simulink model "PX4_Run_Mode_R2017b"  (R2017b)
settings: Solver=FixedStepDiscrete  StartTime=0.0  StopTime=10.0  RelTol=1e-3  EnableMultiTasking=on
InitFcn:
  | run('InitFcn_R2017b_no_csc.m');
values from neighbouring files (symbols this model uses):
  A = Pixhawk_CSC.Parameter( {single([diag([1 1 1]) Ts*diag([1 1 1]); diag([0 0 0]) diag([1 1 1])]),'A'} )    [InitFcn.m]    (also in InitFcn_R2016b.m; InitFcn_R2017b_no_csc.m = single([diag([1 1 1]) Ts*diag([1 1 1]); diag([0 0 0]) diag([)
  app = Pixhawk_CSC.Parameter({single( [0.05; 0.05; 0.05]),'app'} )    [InitFcn.m]    (also in InitFcn_R2016b.m; InitFcn_R2017b_no_csc.m = single( [0.05; 0.05; 0.05]))
  B = Pixhawk_CSC.Parameter( {single([Ts^2/2*diag([1 1 1]); Ts*diag([1 1 1])]),'B'} )    [InitFcn.m]    (also in InitFcn_R2016b.m; InitFcn_R2017b_no_csc.m = single([Ts^2/2*diag([1 1 1]); Ts*diag([1 1 1])]))
  Beta = Pixhawk_CSC.Parameter({single( 0.02),'Beta'} )    [InitFcn.m]    (also in InitFcn_R2016b.m; InitFcn_R2017b_no_csc.m = single( 0.02))
  C = Pixhawk_CSC.Parameter( {single([diag([1 1 1]) 0*diag([1 1 1]); zeros(1,2) 1 zeros(1,3)]),'C'} )    [InitFcn.m]    (also in InitFcn_R2016b.m; InitFcn_R2017b_no_csc.m = single([diag([1 1 1]) 0*diag([1 1 1]); zeros(1,2) 1 zeros(1,)
  C1 = Pixhawk_CSC.Parameter({single( 1.08680),'C1'} )    [InitFcn.m]    (also in InitFcn_R2016b.m; InitFcn_R2017b_no_csc.m = single( 1.08680))
  C10 = Pixhawk_CSC.Parameter({single( 0.0000),'C10'} )    [InitFcn.m]    (also in InitFcn_R2016b.m; InitFcn_R2017b_no_csc.m = single( 0.0000))
  C11 = Pixhawk_CSC.Parameter({single(-0.2300),'C11'} )    [InitFcn.m]    (also in InitFcn_R2016b.m; InitFcn_R2017b_no_csc.m = single(-0.2300))
  C12 = Pixhawk_CSC.Parameter({single( 0.0000),'C12'} )    [InitFcn.m]    (also in InitFcn_R2016b.m; InitFcn_R2017b_no_csc.m = single( 0.0000))
  C13 = Pixhawk_CSC.Parameter({single( 0.8000),'C13'} )    [InitFcn.m]    (also in InitFcn_R2016b.m; InitFcn_R2017b_no_csc.m = single( 0.8000))
  C14 = Pixhawk_CSC.Parameter({single( 0.8000),'C14'} )    [InitFcn.m]    (also in InitFcn_R2016b.m; InitFcn_R2017b_no_csc.m = single( 0.8000))
  C15 = Pixhawk_CSC.Parameter({single( 1.73200),'C15'} )    [InitFcn.m]    (also in InitFcn_R2016b.m; InitFcn_R2017b_no_csc.m = single( 1.73200))
  C16 = Pixhawk_CSC.Parameter({single( 0.1000),'C16'} )    [InitFcn.m]    (also in InitFcn_R2016b.m; InitFcn_R2017b_no_csc.m = single( 0.1000))
  C17 = Pixhawk_CSC.Parameter({single( 0.1000),'C17'} )    [InitFcn.m]    (also in InitFcn_R2016b.m; InitFcn_R2017b_no_csc.m = single( 0.1000))
  C18 = Pixhawk_CSC.Parameter({single( 0.0500),'C18'} )    [InitFcn.m]    (also in InitFcn_R2016b.m; InitFcn_R2017b_no_csc.m = single( 0.0500))
  C19 = Pixhawk_CSC.Parameter({single( 0.6000),'C19'} )    [InitFcn.m]    (also in InitFcn_R2016b.m; InitFcn_R2017b_no_csc.m = single( 0.6000))
  C2 = Pixhawk_CSC.Parameter({single( 1.10468),'C2'} )    [InitFcn.m]    (also in InitFcn_R2016b.m; InitFcn_R2017b_no_csc.m = single( 1.10468))
  C20 = Pixhawk_CSC.Parameter({single( 0.6000),'C20'} )    [InitFcn.m]    (also in InitFcn_R2016b.m; InitFcn_R2017b_no_csc.m = single( 0.6000))
  C21 = Pixhawk_CSC.Parameter({single( 1.04558),'C21'} )    [InitFcn.m]    (also in InitFcn_R2016b.m; InitFcn_R2017b_no_csc.m = single( 1.04558))
  C22 = Pixhawk_CSC.Parameter({single( 0.0000),'C22'} )    [InitFcn.m]    (also in InitFcn_R2016b.m; InitFcn_R2017b_no_csc.m = single( 0.0000))
  C23 = Pixhawk_CSC.Parameter({single( 0.0000),'C23'} )    [InitFcn.m]    (also in InitFcn_R2016b.m; InitFcn_R2017b_no_csc.m = single( 0.0000))
  C24 = Pixhawk_CSC.Parameter({single(-11.0000),'C24'} )    [InitFcn.m]    (also in InitFcn_R2016b.m; InitFcn_R2017b_no_csc.m = single(-11.0000))
  C3 = Pixhawk_CSC.Parameter({single( 1.1980),'C3'} )    [InitFcn.m]    (also in InitFcn_R2016b.m; InitFcn_R2017b_no_csc.m = single( 1.1980))
  C4 = Pixhawk_CSC.Parameter({single( 0.0500),'C4'} )    [InitFcn.m]    (also in InitFcn_R2016b.m; InitFcn_R2017b_no_csc.m = single( 0.0500))
  C5 = Pixhawk_CSC.Parameter({single( 0.0500),'C5'} )    [InitFcn.m]    (also in InitFcn_R2016b.m; InitFcn_R2017b_no_csc.m = single( 0.0500))
  C6 = Pixhawk_CSC.Parameter({single( 0.0500),'C6'} )    [InitFcn.m]    (also in InitFcn_R2016b.m; InitFcn_R2017b_no_csc.m = single( 0.0500))
  C7 = Pixhawk_CSC.Parameter({single( 0.35937),'C7'} )    [InitFcn.m]    (also in InitFcn_R2016b.m; InitFcn_R2017b_no_csc.m = single( 0.35937))
  C8 = Pixhawk_CSC.Parameter({single( 0.36528),'C8'} )    [InitFcn.m]    (also in InitFcn_R2016b.m; InitFcn_R2017b_no_csc.m = single( 0.36528))
  C9 = Pixhawk_CSC.Parameter({single( 0.53311),'C9'} )    [InitFcn.m]    (also in InitFcn_R2016b.m; InitFcn_R2017b_no_csc.m = single( 0.53311))
  C_1 = Pixhawk_CSC.Parameter( {single([diag([1 1 1]) 0*diag([1 1 1])]),'C1'} )    [InitFcn.m]    (also in InitFcn_R2016b.m; InitFcn_R2017b_no_csc.m = single([diag([1 1 1]) 0*diag([1 1 1])]))
  CAL_ACC0_XOFFSET = Pixhawk_CSC.Parameter( {single( 0.122052  ),'CAL_ACC0_XOFFSET'} )    [InitFcn.m]    (also in InitFcn_R2016b.m; InitFcn_R2017b_no_csc.m = single( 0.122052  ))
  CAL_ACC0_XXSCALE = Pixhawk_CSC.Parameter( {single(  1.01218    ),'CAL_ACC0_XXSCALE'} )    [InitFcn.m]    (also in InitFcn_R2016b.m; InitFcn_R2017b_no_csc.m = single(  1.01218    ))
  CAL_ACC0_XYSCALE = Pixhawk_CSC.Parameter( {single( -0.00443301 ),'CAL_ACC0_XYSCALE'} )    [InitFcn.m]    (also in InitFcn_R2016b.m; InitFcn_R2017b_no_csc.m = single( -0.00443301 ))
  CAL_ACC0_XZSCALE = Pixhawk_CSC.Parameter( {single( -0.00505793 ),'CAL_ACC0_XZSCALE'} )    [InitFcn.m]    (also in InitFcn_R2016b.m; InitFcn_R2017b_no_csc.m = single( -0.00505793 ))
  CAL_ACC0_YOFFSET = Pixhawk_CSC.Parameter( {single( 0.00281205),'CAL_ACC0_YOFFSET'} )    [InitFcn.m]    (also in InitFcn_R2016b.m; InitFcn_R2017b_no_csc.m = single( 0.00281205))
  CAL_ACC0_YXSCALE = Pixhawk_CSC.Parameter( {single( -0.00443301 ),'CAL_ACC0_YXSCALE'} )    [InitFcn.m]    (also in InitFcn_R2016b.m; InitFcn_R2017b_no_csc.m = single( -0.00443301 ))
  CAL_ACC0_YYSCALE = Pixhawk_CSC.Parameter( {single(  1.00234    ),'CAL_ACC0_YYSCALE'} )    [InitFcn.m]    (also in InitFcn_R2016b.m; InitFcn_R2017b_no_csc.m = single(  1.00234    ))
  CAL_ACC0_YZSCALE = Pixhawk_CSC.Parameter( {single(  0.0160883  ),'CAL_ACC0_YZSCALE'} )    [InitFcn.m]    (also in InitFcn_R2016b.m; InitFcn_R2017b_no_csc.m = single(  0.0160883  ))
  CAL_ACC0_ZOFFSET = Pixhawk_CSC.Parameter( {single(-0.0298121 ),'CAL_ACC0_ZOFFSET'} )    [InitFcn.m]    (also in InitFcn_R2016b.m; InitFcn_R2017b_no_csc.m = single(-0.0298121 ))
  CAL_ACC0_ZXSCALE = Pixhawk_CSC.Parameter( {single( -0.00505793 ),'CAL_ACC0_ZXSCALE'} )    [InitFcn.m]    (also in InitFcn_R2016b.m; InitFcn_R2017b_no_csc.m = single( -0.00505793 ))
  CAL_ACC0_ZYSCALE = Pixhawk_CSC.Parameter( {single(  0.0160883  ),'CAL_ACC0_ZYSCALE'} )    [InitFcn.m]    (also in InitFcn_R2016b.m; InitFcn_R2017b_no_csc.m = single(  0.0160883  ))
  CAL_ACC0_ZZSCALE = Pixhawk_CSC.Parameter( {single(  0.983604   ),'CAL_ACC0_ZZSCALE'} )    [InitFcn.m]    (also in InitFcn_R2016b.m; InitFcn_R2017b_no_csc.m = single(  0.983604   ))
  CAL_BAR_OFFSET = Pixhawk_CSC.Parameter( {single( -20.8468),'CAL_BAR_OFFSET'} )    [InitFcn.m]    (also in InitFcn_R2016b.m; InitFcn_R2017b_no_csc.m = single( -20.8468))
  CAL_BAR_SCALE = Pixhawk_CSC.Parameter( {single(   1.0632),'CAL_BAR_SCALE'} )    [InitFcn.m]    (also in InitFcn_R2016b.m; InitFcn_R2017b_no_csc.m = single(   1.0632))
  CAL_BAT0_XOFFSET = Pixhawk_CSC.Parameter( {single( 0.0000),'CAL_BAT0_XOFFSET'} )    [InitFcn.m]    (also in InitFcn_R2016b.m; InitFcn_R2017b_no_csc.m = single( 0.0000))
  CAL_BAT0_XXSCALE = Pixhawk_CSC.Parameter( {single(  1.0000),'CAL_BAT0_XXSCALE'} )    [InitFcn.m]    (also in InitFcn_R2016b.m; InitFcn_R2017b_no_csc.m = single(  1.0000))
  CAL_BAT0_XYSCALE = Pixhawk_CSC.Parameter( {single(  0.0000),'CAL_BAT0_XYSCALE'} )    [InitFcn.m]    (also in InitFcn_R2016b.m; InitFcn_R2017b_no_csc.m = single(  0.0000))
  CAL_BAT0_XZSCALE = Pixhawk_CSC.Parameter( {single(  0.0000),'CAL_BAT0_XZSCALE'} )    [InitFcn.m]    (also in InitFcn_R2016b.m; InitFcn_R2017b_no_csc.m = single(  0.0000))
  CAL_BAT0_YOFFSET = Pixhawk_CSC.Parameter( {single( 0.0000),'CAL_BAT0_YOFFSET'} )    [InitFcn.m]    (also in InitFcn_R2016b.m; InitFcn_R2017b_no_csc.m = single( 0.0000))
  CAL_BAT0_YXSCALE = Pixhawk_CSC.Parameter( {single(  0.0000),'CAL_BAT0_YXSCALE'} )    [InitFcn.m]    (also in InitFcn_R2016b.m; InitFcn_R2017b_no_csc.m = single(  0.0000))
  CAL_BAT0_YYSCALE = Pixhawk_CSC.Parameter( {single(  1.0000),'CAL_BAT0_YYSCALE'} )    [InitFcn.m]    (also in InitFcn_R2016b.m; InitFcn_R2017b_no_csc.m = single(  1.0000))
  CAL_BAT0_YZSCALE = Pixhawk_CSC.Parameter( {single(  0.0000),'CAL_BAT0_YZSCALE'} )    [InitFcn.m]    (also in InitFcn_R2016b.m; InitFcn_R2017b_no_csc.m = single(  0.0000))
  CAL_BAT0_ZOFFSET = Pixhawk_CSC.Parameter( {single( 0.0000),'CAL_BAT0_ZOFFSET'} )    [InitFcn.m]    (also in InitFcn_R2016b.m; InitFcn_R2017b_no_csc.m = single( 0.0000))
  CAL_BAT0_ZXSCALE = Pixhawk_CSC.Parameter( {single(  0.0000),'CAL_BAT0_ZXSCALE'} )    [InitFcn.m]    (also in InitFcn_R2016b.m; InitFcn_R2017b_no_csc.m = single(  0.0000))
  CAL_BAT0_ZYSCALE = Pixhawk_CSC.Parameter( {single(  0.0000),'CAL_BAT0_ZYSCALE'} )    [InitFcn.m]    (also in InitFcn_R2016b.m; InitFcn_R2017b_no_csc.m = single(  0.0000))
  CAL_BAT0_ZZSCALE = Pixhawk_CSC.Parameter( {single(  1.0000),'CAL_BAT0_ZZSCALE'} )    [InitFcn.m]    (also in InitFcn_R2016b.m; InitFcn_R2017b_no_csc.m = single(  1.0000))
  CAL_GPS0_XOFFSET = Pixhawk_CSC.Parameter( {single( 0.0000),'CAL_GPS0_XOFFSET'} )    [InitFcn.m]    (also in InitFcn_R2016b.m; InitFcn_R2017b_no_csc.m = single( 0.0000))
  CAL_GPS0_XXSCALE = Pixhawk_CSC.Parameter( {single(  0.0100),'CAL_GPS0_XXSCALE'} )    [InitFcn.m]    (also in InitFcn_R2016b.m; InitFcn_R2017b_no_csc.m = single(  0.0100))
  CAL_GPS0_XYSCALE = Pixhawk_CSC.Parameter( {single(  0.0000),'CAL_GPS0_XYSCALE'} )    [InitFcn.m]    (also in InitFcn_R2016b.m; InitFcn_R2017b_no_csc.m = single(  0.0000))
  CAL_GPS0_XZSCALE = Pixhawk_CSC.Parameter( {single(  0.0000),'CAL_GPS0_XZSCALE'} )    [InitFcn.m]    (also in InitFcn_R2016b.m; InitFcn_R2017b_no_csc.m = single(  0.0000))
  CAL_GPS0_YOFFSET = Pixhawk_CSC.Parameter( {single( 0.0000),'CAL_GPS0_YOFFSET'} )    [InitFcn.m]    (also in InitFcn_R2016b.m; InitFcn_R2017b_no_csc.m = single( 0.0000))
  CAL_GPS0_YXSCALE = Pixhawk_CSC.Parameter( {single(  0.0000),'CAL_GPS0_YXSCALE'} )    [InitFcn.m]    (also in InitFcn_R2016b.m; InitFcn_R2017b_no_csc.m = single(  0.0000))
  CAL_GPS0_YYSCALE = Pixhawk_CSC.Parameter( {single(  0.0100),'CAL_GPS0_YYSCALE'} )    [InitFcn.m]    (also in InitFcn_R2016b.m; InitFcn_R2017b_no_csc.m = single(  0.0100))
  CAL_GPS0_YZSCALE = Pixhawk_CSC.Parameter( {single(  0.0000),'CAL_GPS0_YZSCALE'} )    [InitFcn.m]    (also in InitFcn_R2016b.m; InitFcn_R2017b_no_csc.m = single(  0.0000))
  CAL_GPS0_ZOFFSET = Pixhawk_CSC.Parameter( {single( 0.0000),'CAL_GPS0_ZOFFSET'} )    [InitFcn.m]    (also in InitFcn_R2016b.m; InitFcn_R2017b_no_csc.m = single( 0.0000))
  CAL_GPS0_ZXSCALE = Pixhawk_CSC.Parameter( {single(  0.0000),'CAL_GPS0_ZXSCALE'} )    [InitFcn.m]    (also in InitFcn_R2016b.m; InitFcn_R2017b_no_csc.m = single(  0.0000))
  CAL_GPS0_ZYSCALE = Pixhawk_CSC.Parameter( {single(  0.0000),'CAL_GPS0_ZYSCALE'} )    [InitFcn.m]    (also in InitFcn_R2016b.m; InitFcn_R2017b_no_csc.m = single(  0.0000))
  CAL_GPS0_ZZSCALE = Pixhawk_CSC.Parameter( {single( -0.0010),'CAL_GPS0_ZZSCALE'} )    [InitFcn.m]    (also in InitFcn_R2016b.m; InitFcn_R2017b_no_csc.m = single( -0.0010))
  CAL_GYRO0_XXSCALE = Pixhawk_CSC.Parameter( {single(0.992736),'CAL_GYRO0_XXSCALE'} )    [InitFcn.m]    (also in InitFcn_R2016b.m; InitFcn_R2017b_no_csc.m = single(0.992736))
  CAL_GYRO0_XYSCALE = Pixhawk_CSC.Parameter( {single(0.0000),'CAL_GYRO0_XYSCALE'} )    [InitFcn.m]    (also in InitFcn_R2016b.m; InitFcn_R2017b_no_csc.m = single(0.0000))
  CAL_GYRO0_XZSCALE = Pixhawk_CSC.Parameter( {single(0.0000),'CAL_GYRO0_XZSCALE'} )    [InitFcn.m]    (also in InitFcn_R2016b.m; InitFcn_R2017b_no_csc.m = single(0.0000))
  CAL_GYRO0_YXSCALE = Pixhawk_CSC.Parameter( {single(0.0000),'CAL_GYRO0_YXSCALE'} )    [InitFcn.m]    (also in InitFcn_R2016b.m; InitFcn_R2017b_no_csc.m = single(0.0000))
  CAL_GYRO0_YYSCALE = Pixhawk_CSC.Parameter( {single(1.01609),'CAL_GYRO0_YYSCALE'} )    [InitFcn.m]    (also in InitFcn_R2016b.m; InitFcn_R2017b_no_csc.m = single(1.01609))
  CAL_GYRO0_YZSCALE = Pixhawk_CSC.Parameter( {single(0.0000),'CAL_GYRO0_YZSCALE'} )    [InitFcn.m]    (also in InitFcn_R2016b.m; InitFcn_R2017b_no_csc.m = single(0.0000))
  CAL_GYRO0_ZXSCALE = Pixhawk_CSC.Parameter( {single(0.0000),'CAL_GYRO0_ZXSCALE'} )    [InitFcn.m]    (also in InitFcn_R2016b.m; InitFcn_R2017b_no_csc.m = single(0.0000))
  CAL_GYRO0_ZYSCALE = Pixhawk_CSC.Parameter( {single(0.0000),'CAL_GYRO0_ZYSCALE'} )    [InitFcn.m]    (also in InitFcn_R2016b.m; InitFcn_R2017b_no_csc.m = single(0.0000))
  CAL_GYRO0_ZZSCALE = Pixhawk_CSC.Parameter( {single(1.03003),'CAL_GYRO0_ZZSCALE'} )    [InitFcn.m]    (also in InitFcn_R2016b.m; InitFcn_R2017b_no_csc.m = single(1.03003))
  CAL_MAG0_XCURCOR = Pixhawk_CSC.Parameter( {single( 0.0017     ),'CAL_MAG0_XCURCOR'} )    [InitFcn.m]    (also in InitFcn_R2016b.m; InitFcn_R2017b_no_csc.m = single( 0.0017     ))
  CAL_MAG0_XOFFSET = Pixhawk_CSC.Parameter( {single( 0.0446372  ),'CAL_MAG0_XOFFSET'} )    [InitFcn.m]    (also in InitFcn_R2016b.m; InitFcn_R2017b_no_csc.m = single( 0.0446372  ))
  CAL_MAG0_XXSCALE = Pixhawk_CSC.Parameter( {single(  1.01563   ),'CAL_MAG0_XXSCALE'} )    [InitFcn.m]    (also in InitFcn_R2016b.m; InitFcn_R2017b_no_csc.m = single(  1.01563   ))
  CAL_MAG0_XYSCALE = Pixhawk_CSC.Parameter( {single( -0.0612061 ),'CAL_MAG0_XYSCALE'} )    [InitFcn.m]    (also in InitFcn_R2016b.m; InitFcn_R2017b_no_csc.m = single( -0.0612061 ))
  CAL_MAG0_XZSCALE = Pixhawk_CSC.Parameter( {single( -0.011532  ),'CAL_MAG0_XZSCALE'} )    [InitFcn.m]    (also in InitFcn_R2016b.m; InitFcn_R2017b_no_csc.m = single( -0.011532  ))
  CAL_MAG0_YCURCOR = Pixhawk_CSC.Parameter( {single(-0.0075     ),'CAL_MAG0_YCURCOR'} )    [InitFcn.m]    (also in InitFcn_R2016b.m; InitFcn_R2017b_no_csc.m = single(-0.0075     ))
  CAL_MAG0_YOFFSET = Pixhawk_CSC.Parameter( {single( 0.0700776  ),'CAL_MAG0_YOFFSET'} )    [InitFcn.m]    (also in InitFcn_R2016b.m; InitFcn_R2017b_no_csc.m = single( 0.0700776  ))
  CAL_MAG0_YXSCALE = Pixhawk_CSC.Parameter( {single( -0.0612061 ),'CAL_MAG0_YXSCALE'} )    [InitFcn.m]    (also in InitFcn_R2016b.m; InitFcn_R2017b_no_csc.m = single( -0.0612061 ))
  CAL_MAG0_YYSCALE = Pixhawk_CSC.Parameter( {single(  1.00593   ),'CAL_MAG0_YYSCALE'} )    [InitFcn.m]    (also in InitFcn_R2016b.m; InitFcn_R2017b_no_csc.m = single(  1.00593   ))
  CAL_MAG0_YZSCALE = Pixhawk_CSC.Parameter( {single(  0.0144582 ),'CAL_MAG0_YZSCALE'} )    [InitFcn.m]    (also in InitFcn_R2016b.m; InitFcn_R2017b_no_csc.m = single(  0.0144582 ))
  CAL_MAG0_ZCURCOR = Pixhawk_CSC.Parameter( {single(-0.0080     ),'CAL_MAG0_ZCURCOR'} )    [InitFcn.m]    (also in InitFcn_R2016b.m; InitFcn_R2017b_no_csc.m = single(-0.0080     ))
  CAL_MAG0_ZOFFSET = Pixhawk_CSC.Parameter( {single( 0.00201742 ),'CAL_MAG0_ZOFFSET'} )    [InitFcn.m]    (also in InitFcn_R2016b.m; InitFcn_R2017b_no_csc.m = single( 0.00201742 ))
  CAL_MAG0_ZXSCALE = Pixhawk_CSC.Parameter( {single( -0.011532  ),'CAL_MAG0_ZXSCALE'} )    [InitFcn.m]    (also in InitFcn_R2016b.m; InitFcn_R2017b_no_csc.m = single( -0.011532  ))
  CAL_MAG0_ZYSCALE = Pixhawk_CSC.Parameter( {single(  0.0144582 ),'CAL_MAG0_ZYSCALE'} )    [InitFcn.m]    (also in InitFcn_R2016b.m; InitFcn_R2017b_no_csc.m = single(  0.0144582 ))
  CAL_MAG0_ZZSCALE = Pixhawk_CSC.Parameter( {single(  0.986813  ),'CAL_MAG0_ZZSCALE'} )    [InitFcn.m]    (also in InitFcn_R2016b.m; InitFcn_R2017b_no_csc.m = single(  0.986813  ))
  CAL_SONAR_OFFSET = Pixhawk_CSC.Parameter( {single( -6.8730),'CAL_SONAR_OFFSET'} )    [InitFcn.m]    (also in InitFcn_R2016b.m; InitFcn_R2017b_no_csc.m = single( -6.8730))
  CAL_SONAR_SCALE = Pixhawk_CSC.Parameter( {single(-438.1875),'CAL_SONAR_SCALE'} )    [InitFcn.m]    (also in InitFcn_R2016b.m; InitFcn_R2017b_no_csc.m = single(-438.1875))
  COM_RATE = double(10)    [InitFcn.m]    (also in InitFcn_R2016b.m; InitFcn_R2017b_no_csc.m)
  D = Pixhawk_CSC.Parameter( {single(zeros(size(C.Value,1), size(B.Value,2))),'D'} )    [InitFcn.m]    (also in InitFcn_R2016b.m; InitFcn_R2017b_no_csc.m = single(zeros(size(C,1), size(B,2))))
  Dip0 = Pixhawk_CSC.Parameter({single( 1.2),'Dip0'} )    [InitFcn.m]    (also in InitFcn_R2016b.m; InitFcn_R2017b_no_csc.m = single( 1.2))
  I = Pixhawk_CSC.Parameter( {single(eye(size(Q.Value))),'I'} )    [InitFcn.m]    (also in InitFcn_R2016b.m; InitFcn_R2017b_no_csc.m = single(eye(size(Q))))
  Jxx = Pixhawk_CSC.Parameter( {single(J(1,1)),'Jxx'} )    [InitFcn.m]    (also in InitFcn_R2016b.m; InitFcn_R2017b_no_csc.m = single(J(1,1)))
  Jyy = Pixhawk_CSC.Parameter( {single(J(2,2)),'Jyy'} )    [InitFcn.m]    (also in InitFcn_R2016b.m; InitFcn_R2017b_no_csc.m = single(J(2,2)))
  Jzz = Pixhawk_CSC.Parameter( {single(J(3,3)),'Jzz'} )    [InitFcn.m]    (also in InitFcn_R2016b.m; InitFcn_R2017b_no_csc.m = single(J(3,3)))
  Kapp = Pixhawk_CSC.Parameter({single( 1.2),'Kapp'} )    [InitFcn.m]    (also in InitFcn_R2016b.m; InitFcn_R2017b_no_csc.m = single( 1.2))
  Kx = Pixhawk_CSC.Parameter({single( Kx),'Kx'} )    [InitFcn.m]    (also in InitFcn_R2016b.m = Pixhawk_CSC.Parameter({single( [0.60 0.9]),'Kx'} ); InitFcn_R2017b_no_csc.m = single( [0.60 0.9]))
  Ky = Pixhawk_CSC.Parameter({single( Ky),'Ky'} )    [InitFcn.m]    (also in InitFcn_R2016b.m = Pixhawk_CSC.Parameter({single( [0.4 0.9]),'Ky'} ); InitFcn_R2017b_no_csc.m = single( [0.4 0.9]))
  LPF_REF_DEN = Pixhawk_CSC.Parameter( {single([1.0000 -0.8187]),'LPF_REF_DEN'} )    [InitFcn.m]    (also in InitFcn_R2016b.m; InitFcn_R2017b_no_csc.m = single([1.0000 -0.8187]))
  LPF_REF_NUM = Pixhawk_CSC.Parameter( {single([0.0000  0.1813]),'LPF_REF_NUM'} )    [InitFcn.m]    (also in InitFcn_R2016b.m; InitFcn_R2017b_no_csc.m = single([0.0000  0.1813]))
  m0 = Pixhawk_CSC.Parameter({single( 0.452857),'m0'} )    [InitFcn.m]    (also in InitFcn_R2016b.m; InitFcn_R2017b_no_csc.m = single( 0.452857))
  mn = [0.01; 0.01; 0.01; 0.01]    [InitFcn.m]    (also in InitFcn_R2016b.m; InitFcn_R2017b_no_csc.m)
  MOV_AVG_WINDOW = Pixhawk_CSC.Parameter( {single(100),'MOV_AVG_WINDOW'} )    [InitFcn.m]    (also in InitFcn_R2016b.m; InitFcn_R2017b_no_csc.m = single(100))
  Ox0 = Pixhawk_CSC.Parameter({single(O_x0),'Ox0'} )    [InitFcn.m]    (also in InitFcn_R2016b.m; InitFcn_R2017b_no_csc.m = single(O_x0))
  Oxa = Pixhawk_CSC.Parameter({single(O_x.a),'Oxa'} )    [InitFcn.m]    (also in InitFcn_R2016b.m; InitFcn_R2017b_no_csc.m = single(O_x.a))
  Oxb = Pixhawk_CSC.Parameter({single(O_x.b),'Oxb'} )    [InitFcn.m]    (also in InitFcn_R2016b.m; InitFcn_R2017b_no_csc.m = single(O_x.b))
  Oxc = Pixhawk_CSC.Parameter({single(O_x.c),'Oxc'} )    [InitFcn.m]    (also in InitFcn_R2016b.m; InitFcn_R2017b_no_csc.m = single(O_x.c))
  Oxd = Pixhawk_CSC.Parameter({single(O_x.d),'Oxd'} )    [InitFcn.m]    (also in InitFcn_R2016b.m; InitFcn_R2017b_no_csc.m = single(O_x.d))
  Oy0 = Pixhawk_CSC.Parameter({single(O_y0),'Oy0'} )    [InitFcn.m]    (also in InitFcn_R2016b.m; InitFcn_R2017b_no_csc.m = single(O_y0))
  Oya = Pixhawk_CSC.Parameter({single(O_y.a),'Oya'} )    [InitFcn.m]    (also in InitFcn_R2016b.m; InitFcn_R2017b_no_csc.m = single(O_y.a))
  Oyb = Pixhawk_CSC.Parameter({single(O_y.b),'Oyb'} )    [InitFcn.m]    (also in InitFcn_R2016b.m; InitFcn_R2017b_no_csc.m = single(O_y.b))
  Oyc = Pixhawk_CSC.Parameter({single(O_y.c),'Oyc'} )    [InitFcn.m]    (also in InitFcn_R2016b.m; InitFcn_R2017b_no_csc.m = single(O_y.c))
  Oyd = Pixhawk_CSC.Parameter({single(O_y.d),'Oyd'} )    [InitFcn.m]    (also in InitFcn_R2016b.m; InitFcn_R2017b_no_csc.m = single(O_y.d))
  Oz0 = Pixhawk_CSC.Parameter({single(O_z0),'Oz0'} )    [InitFcn.m]    (also in InitFcn_R2016b.m; InitFcn_R2017b_no_csc.m = single(O_z0))
  ... (+53 more)
undefined symbols (not defined in the file or in its folder): AccX, AccY, AccZ, Altitude, ax, ay, az, Current, FILTER_N, GPS_TS, GyroX, GyroY, GyroZ, Latitude, Longitude, M1_PWM, M2_PWM, M3_PWM, M4_PWM, MagX, MagY, MagZ, mAH, MOTOR, phi, Position_TS, psi, PX4_TUNE_ENUM, RGBLED_COLOR_ENUM, RGBLED_MODE_ENUM, S_AccX, S_AccY, S_AccZ, S_Altitude, S_Baro, S_Current, S_GyroX, S_GyroY, S_GyroZ, S_Latitude, S_Longitude, S_MagX, S_MagY, S_MagZ, S_mAH, S_N_Sat, S_Voltage, T_PITCH, T_ROLL, T_THROTTLE, theta, v, Voltage, w, wx, wxd, wy, wyd, wz ... (+4)
libraries: simulink x31, pixhawk_slib_sensors_actuators x7, pixhawk_slib_ADC_serial x5, pixhawk_slib_misc_utils x3, etargetslib x2
(part 5 of 7)

== system PX4_Run_Mode_R2017b/SENSOR_FILTER/Fixed Bias removal and scaling/Sonar Calibration ==
  FILTERED_SENSOR_DATA_IN : Inport
  RAW_SENSOR_DATA_IN : Inport  Port=2
  Bus Assignment : BusAssignment  AssignedSignals=Sonar
  Bus Selector2 : BusSelector  OutputSignals=S_Sonar  OutputAsBus=on
  Bus to Vector : BusToVector
  Constant5 : Constant  Value=CAL_SONAR_SCALE  SampleTime=Ts
  Constant6 : Constant  Value=CAL_SONAR_OFFSET  SampleTime=Ts
  MATLAB Function : MATLAB Function  TreatAsAtomicUnit=on
  Mux : Mux  Inputs=2
  Parameters : Outport
  FILTERED_SENSOR_DATA_OUT : Outport  Port=2
  wires:
  FILTERED_SENSOR_DATA_IN/1 -> Bus Assignment/1
  MATLAB Function/1(Sonar_Out) -> Bus Assignment/2
  Bus Assignment/1 -> FILTERED_SENSOR_DATA_OUT/1
  RAW_SENSOR_DATA_IN/1 -> Bus Selector2/1
  Bus Selector2/1 -> Bus to Vector/1
  Bus to Vector/1 -> MATLAB Function/1(Sonar_In)
  Mux/1 -> Parameters/1
  Constant5/1 -> Mux/1
  Constant6/1 -> Mux/2

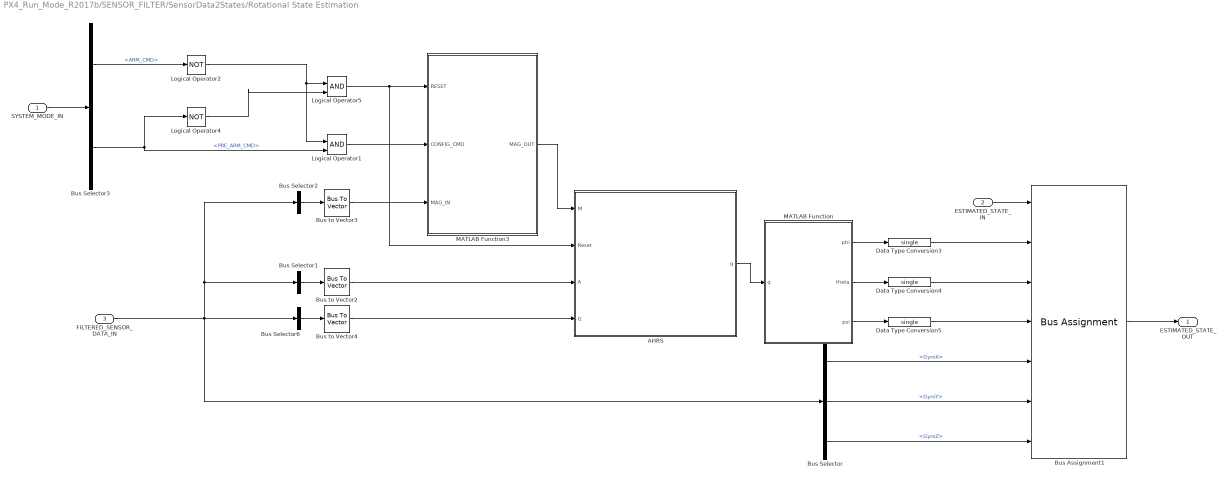
== system PX4_Run_Mode_R2017b/SENSOR_FILTER/SensorData2States/Rotational State Estimation ==
  SYSTEM_MODE_IN : Inport
  ESTIMATED_STATE_IN : Inport  Port=2
  FILTERED_SENSOR_DATA_IN : Inport  Port=3
  AHRS : MATLAB Function  TreatAsAtomicUnit=on
  Bus Assignment1 : BusAssignment  AssignedSignals=phi,theta,psi,wx,wy,wz
  Bus Selector : BusSelector  OutputSignals=GyroX,GyroY,GyroZ
  Bus Selector1 : BusSelector  OutputSignals=AccX,AccY,AccZ  OutputAsBus=on
  Bus Selector2 : BusSelector  OutputSignals=MagX,MagY,MagZ  OutputAsBus=on
  Bus Selector3 : BusSelector  OutputSignals=ARM_CMD,PRE_ARM_CMD
  Bus Selector6 : BusSelector  OutputSignals=GyroX,GyroY,GyroZ  OutputAsBus=on
  Bus to Vector2 : BusToVector
  Bus to Vector3 : BusToVector
  Bus to Vector4 : BusToVector
  Data Type Conversion3 : DataTypeConversion  OutDataTypeStr=single
  Data Type Conversion4 : DataTypeConversion  OutDataTypeStr=single
  Data Type Conversion5 : DataTypeConversion  OutDataTypeStr=single
  Logical Operator1 : Logic  IconShape=distinctive  AllPortsSameDT=off  OutDataTypeStr=boolean
  Logical Operator2 : Logic  Operator=NOT  IconShape=distinctive  AllPortsSameDT=off  OutDataTypeStr=boolean
  Logical Operator4 : Logic  Operator=NOT  IconShape=distinctive  AllPortsSameDT=off  OutDataTypeStr=boolean
  Logical Operator5 : Logic  IconShape=distinctive  AllPortsSameDT=off  OutDataTypeStr=boolean
  MATLAB Function : MATLAB Function  TreatAsAtomicUnit=on
  MATLAB Function3 : MATLAB Function  TreatAsAtomicUnit=on
  ESTIMATED_STATE_OUT : Outport
  wires:
  Bus Assignment1/1 -> ESTIMATED_STATE_OUT/1
  ESTIMATED_STATE_IN/1 -> Bus Assignment1/1
  Bus Selector/2 -> Bus Assignment1/6  "<GyroY>"
  Bus Selector/1 -> Bus Assignment1/5  "<GyroX>"
  Bus Selector/3 -> Bus Assignment1/7  "<GyroZ>"
  FILTERED_SENSOR_DATA_IN/1 -> Bus Selector/1, Bus Selector2/1, Bus Selector1/1, Bus Selector6/1
  Bus to Vector2/1 -> AHRS/3(A)
  Bus Selector1/1 -> Bus to Vector2/1
  Bus to Vector4/1 -> AHRS/4(G)
  Bus Selector6/1 -> Bus to Vector4/1
  Bus Selector2/1 -> Bus to Vector3/1
  AHRS/1(q) -> MATLAB Function/1(q)
  MATLAB Function/3(psi) -> Data Type Conversion5/1
  MATLAB Function/2(theta) -> Data Type Conversion4/1
  MATLAB Function/1(phi) -> Data Type Conversion3/1
  Data Type Conversion3/1 -> Bus Assignment1/2
  Data Type Conversion4/1 -> Bus Assignment1/3
  Data Type Conversion5/1 -> Bus Assignment1/4
  SYSTEM_MODE_IN/1 -> Bus Selector3/1
  Bus Selector3/1 -> Logical Operator2/1  "<ARM_CMD>"
  Logical Operator2/1 -> Logical Operator1/1, Logical Operator5/1
  Bus Selector3/2 -> Logical Operator4/1, Logical Operator1/2  "<PRE_ARM_CMD>"
  Logical Operator5/1 -> AHRS/2(Reset), MATLAB Function3/1(RESET)
  Logical Operator4/1 -> Logical Operator5/2
  Logical Operator1/1 -> MATLAB Function3/2(CONFIG_CMD)
  Bus to Vector3/1 -> MATLAB Function3/3(MAG_IN)
  MATLAB Function3/1(MAG_OUT) -> AHRS/1(M)

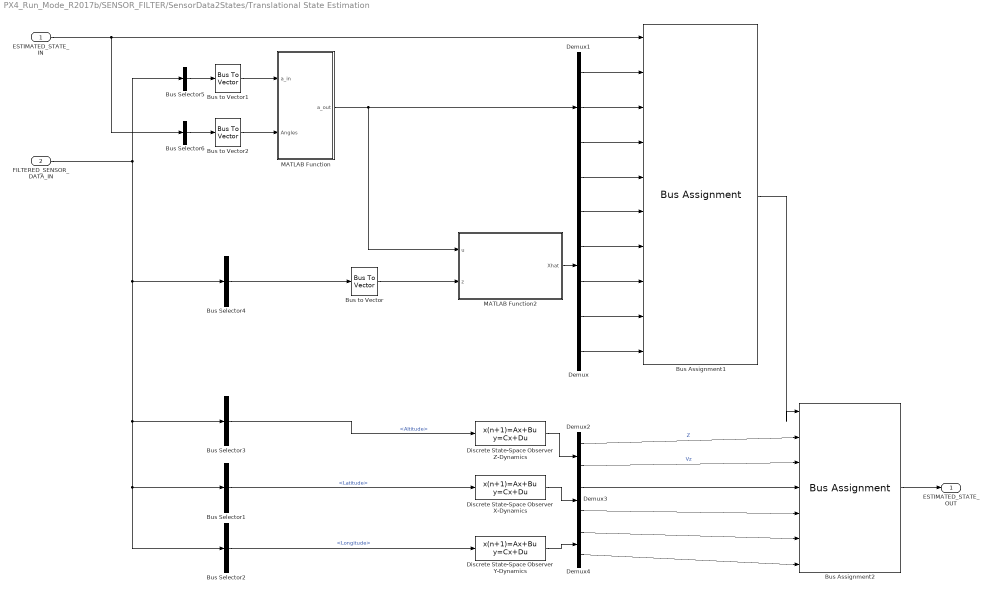
== system PX4_Run_Mode_R2017b/SENSOR_FILTER/SensorData2States/Translational State Estimation ==
  ESTIMATED_STATE_IN : Inport
  FILTERED_SENSOR_DATA_IN : Inport  Port=2
  Bus Assignment1 : BusAssignment  AssignedSignals=ax,ay,az,x,y,z,u,v,w
  Bus Assignment2 : BusAssignment  AssignedSignals=z,w,x,u,y,v
  Bus Selector1 : BusSelector  OutputSignals=Latitude
  Bus Selector2 : BusSelector  OutputSignals=Longitude
  Bus Selector3 : BusSelector  OutputSignals=Altitude
  Bus Selector4 : BusSelector  OutputSignals=Latitude,Longitude,Altitude  OutputAsBus=on
  Bus Selector5 : BusSelector  OutputSignals=AccX,AccY,AccZ  OutputAsBus=on
  Bus Selector6 : BusSelector  OutputSignals=phi,theta,psi  OutputAsBus=on
  Bus to Vector : BusToVector
  Bus to Vector1 : BusToVector
  Bus to Vector2 : BusToVector
  Demux : Demux  Outputs=6
  Demux1 : Demux  Outputs=3
  Demux2 : Demux  Outputs=2
  Demux3 : Demux  Outputs=2
  Demux4 : Demux  Outputs=2
  Discrete State-Space Observer X-Dynamics : DiscreteStateSpace  A=Oxa  B=Oxb  C=Oxc  D=Oxd  InitialCondition=Ox0  SampleTime=Ts
  Discrete State-Space Observer Y-Dynamics : DiscreteStateSpace  A=Oya  B=Oyb  C=Oyc  D=Oyd  InitialCondition=Oy0  SampleTime=Ts
  Discrete State-Space Observer Z-Dynamics : DiscreteStateSpace  A=Oza  B=Ozb  C=Ozc  D=Ozd  InitialCondition=Oz0  SampleTime=Ts
  MATLAB Function : MATLAB Function  TreatAsAtomicUnit=on
  MATLAB Function2 : MATLAB Function  TreatAsAtomicUnit=on
  ESTIMATED_STATE_OUT : Outport
  wires:
  ESTIMATED_STATE_IN/1 -> Bus Selector6/1, Bus Assignment1/1
  Bus Assignment1/1 -> Bus Assignment2/1
  Bus to Vector/1 -> MATLAB Function2/2(z)
  Bus Selector4/1 -> Bus to Vector/1
  MATLAB Function2/1(Xhat) -> Demux/1
  Demux/2 -> Bus Assignment1/6
  Demux/3 -> Bus Assignment1/7
  Demux/1 -> Bus Assignment1/5
  Demux/4 -> Bus Assignment1/8
  Demux/5 -> Bus Assignment1/9
  Demux/6 -> Bus Assignment1/10
  Bus to Vector1/1 -> MATLAB Function/1(a_in)
  FILTERED_SENSOR_DATA_IN/1 -> Bus Selector2/1, Bus Selector1/1, Bus Selector3/1, Bus Selector4/1, Bus Selector5/1
  Bus Selector5/1 -> Bus to Vector1/1
  Bus to Vector2/1 -> MATLAB Function/2(Angles)
  Bus Selector6/1 -> Bus to Vector2/1
  MATLAB Function/1(a_out) -> Demux1/1, MATLAB Function2/1(u)
  Demux1/1 -> Bus Assignment1/2
  Demux1/2 -> Bus Assignment1/3
  Demux1/3 -> Bus Assignment1/4
  Bus Selector3/1 -> Discrete State-Space Observer Z-Dynamics/1  "<Altitude>"
  Discrete State-Space Observer Z-Dynamics/1 -> Demux2/1
  Demux2/1 -> Bus Assignment2/2  "Z"
  Demux2/2 -> Bus Assignment2/3  "Vz"
  Bus Assignment2/1 -> ESTIMATED_STATE_OUT/1
  Bus Selector1/1 -> Discrete State-Space Observer X-Dynamics/1  "<Latitude>"
  Bus Selector2/1 -> Discrete State-Space Observer Y-Dynamics/1  "<Longitude>"
  Discrete State-Space Observer X-Dynamics/1 -> Demux3/1
  Discrete State-Space Observer Y-Dynamics/1 -> Demux4/1
  Demux3/1 -> Bus Assignment2/4
  Demux3/2 -> Bus Assignment2/5
  Demux4/1 -> Bus Assignment2/6
  Demux4/2 -> Bus Assignment2/7

== system PX4_Run_Mode_R2017b/SENSOR_FILTER/Fixed Bias removal and scaling/Parameter Bus Creation/Accelerometer ==
  Parameters Accelerometer : Inport
  Bus Creator3 : BusCreator  Inputs=12
  Demux1 : Demux  Outputs=12
  Accelerometer Parameters Out : Outport
  wires:
  Demux1/2 -> Bus Creator3/2  "CAL_ACC0_XYSCALE"
  Demux1/1 -> Bus Creator3/1  "CAL_ACC0_XXSCALE"
  Demux1/6 -> Bus Creator3/6  "CAL_ACC0_YZSCALE"
  Bus Creator3/1 -> Accelerometer Parameters Out/1  "Accelerometer Parameters"
  Demux1/8 -> Bus Creator3/8  "CAL_ACC0_ZYSCALE"
  Demux1/10 -> Bus Creator3/10  "CAL_ACC0_XOFFSET"
  Demux1/9 -> Bus Creator3/9  "CAL_ACC0_ZZSCALE"
  Demux1/5 -> Bus Creator3/5  "CAL_ACC0_YYSCALE"
  Demux1/3 -> Bus Creator3/3  "CAL_ACC0_XZSCALE"
  Demux1/7 -> Bus Creator3/7  "CAL_ACC0_ZXSCALE"
  Demux1/12 -> Bus Creator3/12  "CAL_ACC0_ZOFFSET"
  Demux1/11 -> Bus Creator3/11  "CAL_ACC0_YOFFSET"
  Demux1/4 -> Bus Creator3/4  "CAL_ACC0_YXSCALE"
  Parameters Accelerometer/1 -> Demux1/1

== system PX4_Run_Mode_R2017b/SENSOR_FILTER/Fixed Bias removal and scaling/Parameter Bus Creation/Barometer ==
  Parameters Barometer : Inport
  Bus Creator7 : BusCreator  Inputs=2
  Demux16 : Demux  Outputs=2
  Barometer Parameters Out : Outport
  wires:
  Demux16/2 -> Bus Creator7/2  "CAL_BAR_OFFSET"
  Demux16/1 -> Bus Creator7/1  "CAL_BAR_SCALE"
  Parameters Barometer/1 -> Demux16/1
  Bus Creator7/1 -> Barometer Parameters Out/1  "Barometer Parameters"

== system PX4_Run_Mode_R2017b/SENSOR_FILTER/Fixed Bias removal and scaling/Parameter Bus Creation/Battery ==
  Parameters Battery : Inport
  Bus Creator6 : BusCreator  Inputs=12
  Demux4 : Demux  Outputs=12
  "Battery Parameters Out " : Outport
  wires:
  Demux4/9 -> Bus Creator6/9  "CAL_BAT0_ZZSCALE"
  Demux4/7 -> Bus Creator6/7  "CAL_BAT0_ZXSCALE"
  Demux4/10 -> Bus Creator6/10  "CAL_BAT0_XOFFSET"
  Demux4/5 -> Bus Creator6/5  "CAL_BAT0_YYSCALE"
  Demux4/8 -> Bus Creator6/8  "CAL_BAT0_ZYSCALE"
  Demux4/12 -> Bus Creator6/12  "CAL_BAT0_ZOFFSET"
  Demux4/3 -> Bus Creator6/3  "CAL_BAT0_XZSCALE"
  Demux4/1 -> Bus Creator6/1  "CAL_BAT0_XXSCALE"
  Demux4/11 -> Bus Creator6/11  "CAL_BAT0_YOFFSET"
  Demux4/2 -> Bus Creator6/2  "CAL_BAT0_XYSCALE"
  Demux4/4 -> Bus Creator6/4  "CAL_BAT0_YXSCALE"
  Demux4/6 -> Bus Creator6/6  "CAL_BAT0_YZSCALE"
  Parameters Battery/1 -> Demux4/1
  Bus Creator6/1 -> "Battery Parameters Out "/1  "Battery Parameters"

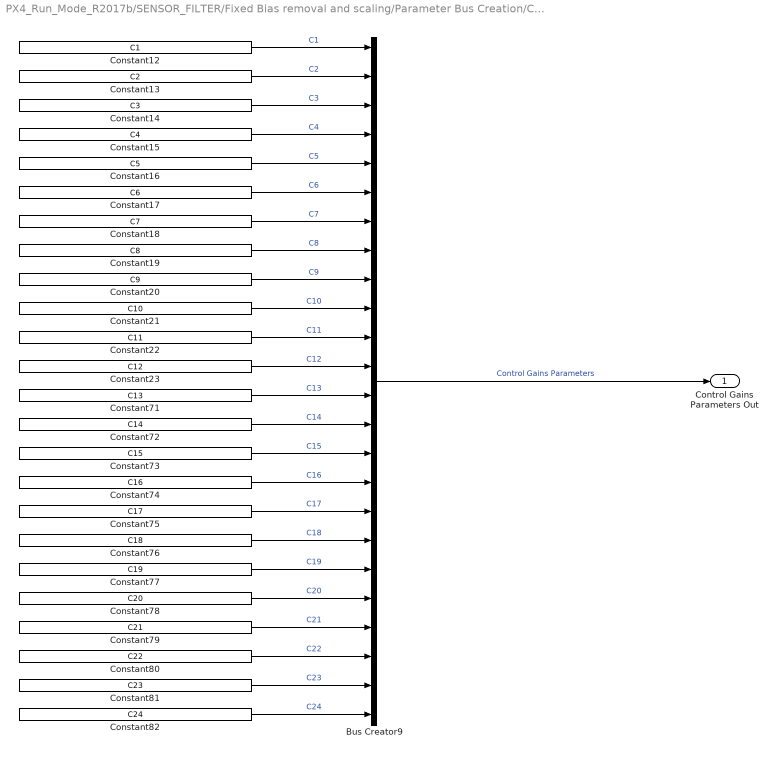
== system PX4_Run_Mode_R2017b/SENSOR_FILTER/Fixed Bias removal and scaling/Parameter Bus Creation/Control Gains ==
  Bus Creator9 : BusCreator  Inputs=24
  Constant12 : Constant  Value=C1  SampleTime=Ts
  Constant13 : Constant  Value=C2  SampleTime=Ts
  Constant14 : Constant  Value=C3  SampleTime=Ts
  Constant15 : Constant  Value=C4  SampleTime=Ts
  Constant16 : Constant  Value=C5  SampleTime=Ts
  Constant17 : Constant  Value=C6  SampleTime=Ts
  Constant18 : Constant  Value=C7  SampleTime=Ts
  Constant19 : Constant  Value=C8  SampleTime=Ts
  Constant20 : Constant  Value=C9  SampleTime=Ts
  Constant21 : Constant  Value=C10  SampleTime=Ts
  Constant22 : Constant  Value=C11  SampleTime=Ts
  Constant23 : Constant  Value=C12  SampleTime=Ts
  Constant71 : Constant  Value=C13  SampleTime=Ts
  Constant72 : Constant  Value=C14  SampleTime=Ts
  Constant73 : Constant  Value=C15  SampleTime=Ts
  Constant74 : Constant  Value=C16  SampleTime=Ts
  Constant75 : Constant  Value=C17  SampleTime=Ts
  Constant76 : Constant  Value=C18  SampleTime=Ts
  Constant77 : Constant  Value=C19  SampleTime=Ts
  Constant78 : Constant  Value=C20  SampleTime=Ts
  Constant79 : Constant  Value=C21  SampleTime=Ts
  Constant80 : Constant  Value=C22  SampleTime=Ts
  Constant81 : Constant  Value=C23  SampleTime=Ts
  Constant82 : Constant  Value=C24  SampleTime=Ts
  Control Gains Parameters Out : Outport
  wires:
  Constant74/1 -> Bus Creator9/16  "C16"
  Constant79/1 -> Bus Creator9/21  "C21"
  Constant77/1 -> Bus Creator9/19  "C19"
  Constant73/1 -> Bus Creator9/15  "C15"
  Constant18/1 -> Bus Creator9/7  "C7"
  Constant81/1 -> Bus Creator9/23  "C23"
  Constant80/1 -> Bus Creator9/22  "C22"
  Constant76/1 -> Bus Creator9/18  "C18"
  Constant13/1 -> Bus Creator9/2  "C2"
  Constant15/1 -> Bus Creator9/4  "C4"
  Constant16/1 -> Bus Creator9/5  "C5"
  Constant75/1 -> Bus Creator9/17  "C17"
  Constant72/1 -> Bus Creator9/14  "C14"
  Constant14/1 -> Bus Creator9/3  "C3"
  Constant17/1 -> Bus Creator9/6  "C6"
  Constant22/1 -> Bus Creator9/11  "C11"
  Constant12/1 -> Bus Creator9/1  "C1"
  Constant21/1 -> Bus Creator9/10  "C10"
  Constant78/1 -> Bus Creator9/20  "C20"
  Constant20/1 -> Bus Creator9/9  "C9"
  Constant23/1 -> Bus Creator9/12  "C12"
  Constant71/1 -> Bus Creator9/13  "C13"
  Constant82/1 -> Bus Creator9/24  "C24"
  Constant19/1 -> Bus Creator9/8  "C8"
  Bus Creator9/1 -> Control Gains Parameters Out/1  "Control Gains Parameters"

== system PX4_Run_Mode_R2017b/SENSOR_FILTER/Fixed Bias removal and scaling/Parameter Bus Creation/Filters ==
  Bus Creator8 : BusCreator  Inputs=4
  Constant10 : Constant  Value=LPF_REF_NUM  SampleTime=Ts
  Constant11 : Constant  Value=LPF_REF_DEN  SampleTime=Ts
  Demux10 : Demux  Outputs=2
  Demux9 : Demux  Outputs=2
  Filter Parameters Out : Outport
  wires:
  Constant11/1 -> Demux10/1
  Constant10/1 -> Demux9/1
  Bus Creator8/1 -> Filter Parameters Out/1  "Filter Parameters"
  Demux9/1 -> Bus Creator8/1  "LPF_REF_NUM_1"
  Demux9/2 -> Bus Creator8/2  "LPF_REF_NUM_2"
  Demux10/1 -> Bus Creator8/3  "LPF_REF_DEN_1"
  Demux10/2 -> Bus Creator8/4  "LPF_REF_DEN_2"

== system PX4_Run_Mode_R2017b/SENSOR_FILTER/Fixed Bias removal and scaling/Parameter Bus Creation/GPS ==
  Parameters GPS : Inport
  Bus Creator5 : BusCreator  Inputs=12
  Demux3 : Demux  Outputs=12
  GPS Parameters Out : Outport
  wires:
  Demux3/3 -> Bus Creator5/3  "CAL_GPS0_XZSCALE"
  Demux3/7 -> Bus Creator5/7  "CAL_GPS0_ZXSCALE"
  Demux3/4 -> Bus Creator5/4  "CAL_GPS0_YXSCALE"
  Demux3/10 -> Bus Creator5/10  "CAL_GPS0_XOFFSET"
  Demux3/9 -> Bus Creator5/9  "CAL_GPS0_ZZSCALE"
  Demux3/5 -> Bus Creator5/5  "CAL_GPS0_YYSCALE"
  Demux3/6 -> Bus Creator5/6  "CAL_GPS0_YZSCALE"
  Demux3/8 -> Bus Creator5/8  "CAL_GPS0_ZYSCALE"
  Demux3/1 -> Bus Creator5/1  "CAL_GPS0_XXSCALE"
  Demux3/12 -> Bus Creator5/12  "CAL_GPS0_ZOFFSET"
  Demux3/11 -> Bus Creator5/11  "CAL_GPS0_YOFFSET"
  Demux3/2 -> Bus Creator5/2  "CAL_GPS0_XYSCALE"
  Parameters GPS/1 -> Demux3/1
  Bus Creator5/1 -> GPS Parameters Out/1  "GPS Parameters"

== system PX4_Run_Mode_R2017b/SENSOR_FILTER/Fixed Bias removal and scaling/Parameter Bus Creation/General Settings ==
  Bus Creator1 : BusCreator  Inputs=6
  Constant1 : Constant  Value=Jyy  SampleTime=Ts
  Constant2 : Constant  Value=Jxx  SampleTime=Ts
  Constant3 : Constant  Value=MOV_AVG_WINDOW  SampleTime=Ts
  Constant4 : Constant  Value=Jzz  SampleTime=Ts
  Constant5 : Constant  Value=Ts  SampleTime=Ts
  Constant6 : Constant  Commented=on  Value=FILTER_N  SampleTime=Ts
  Constant65 : Constant  Value=0  SampleTime=Ts
  Data Type Conversion : DataTypeConversion  OutDataTypeStr=single
  Data Type Conversion1 : DataTypeConversion  OutDataTypeStr=single
  General Parameters Out : Outport
  wires:
  Constant4/1 -> Bus Creator1/6  "Jzz"
  Constant1/1 -> Bus Creator1/5  "Jyy"
  Constant2/1 -> Bus Creator1/4  "Jxx"
  Constant5/1 -> Data Type Conversion/1  "Ts"
  Constant3/1 -> Bus Creator1/2  "MOV_AVG_WINDOW"
  Data Type Conversion/1 -> Bus Creator1/1  "Ts"
  Constant65/1 -> Data Type Conversion1/1  "FILTER_N"
  Bus Creator1/1 -> General Parameters Out/1  "General Parameters"
  Data Type Conversion1/1 -> Bus Creator1/3  "FILTER_N"

== system PX4_Run_Mode_R2017b/SENSOR_FILTER/Fixed Bias removal and scaling/Parameter Bus Creation/Gyroscope ==
  Parameters Gyroscope : Inport
  Bus Creator4 : BusCreator  Inputs=12
  Demux2 : Demux  Outputs=12
  Gyroscope Parameters Out : Outport
  wires:
  Demux2/4 -> Bus Creator4/4  "CAL_GYRO0_YXSCALE"
  Demux2/2 -> Bus Creator4/2  "CAL_GYRO0_XYSCALE"
  Demux2/8 -> Bus Creator4/8  "CAL_GYRO0_ZYSCALE"
  Demux2/10 -> Bus Creator4/10  "CAL_GYRO0_XOFFSET"
  Demux2/12 -> Bus Creator4/12  "CAL_GYRO0_ZOFFSET"
  Demux2/3 -> Bus Creator4/3  "CAL_GYRO0_XZSCALE"
  Demux2/5 -> Bus Creator4/5  "CAL_GYRO0_YYSCALE"
  Demux2/6 -> Bus Creator4/6  "CAL_GYRO0_YZSCALE"
  Demux2/9 -> Bus Creator4/9  "CAL_GYRO0_ZZSCALE"
  Demux2/1 -> Bus Creator4/1  "CAL_GYRO0_XXSCALE"
  Demux2/11 -> Bus Creator4/11  "CAL_GYRO0_YOFFSET"
  Demux2/7 -> Bus Creator4/7  "CAL_GYRO0_ZXSCALE"
  Parameters Gyroscope/1 -> Demux2/1
  Bus Creator4/1 -> Gyroscope Parameters Out/1  "Gyroscope Parameters"

== system PX4_Run_Mode_R2017b/SENSOR_FILTER/Fixed Bias removal and scaling/Parameter Bus Creation/Initial State Bias ==
  Bus Creator14 : BusCreator  Inputs=18
  Demux11 : Demux  Outputs=18
  Initiate_State_Bias : MATLAB Function  TreatAsAtomicUnit=on
  State Bias Parameters Out : Outport
  wires:
  Initiate_State_Bias/1(BIAS_STATE) -> Demux11/1
  Demux11/12 -> Bus Creator14/12  "WZ_BIAS"
  Demux11/1 -> Bus Creator14/1  "X_BIAS"
  Demux11/15 -> Bus Creator14/15  "AZ_BIAS"
  Demux11/4 -> Bus Creator14/4  "PHI_BIAS"
  Demux11/9 -> Bus Creator14/9  "W_BIAS"
  Demux11/7 -> Bus Creator14/7  "U_BIAS"
  Demux11/11 -> Bus Creator14/11  "WY_BIAS"
  Demux11/13 -> Bus Creator14/13  "AX_BIAS"
  Demux11/18 -> Bus Creator14/18  "WZD_BIAS"
  Bus Creator14/1 -> State Bias Parameters Out/1  "State Bias Parameters"
  Demux11/3 -> Bus Creator14/3  "Z_BIAS"
  Demux11/5 -> Bus Creator14/5  "THETA_BIAS"
  Demux11/8 -> Bus Creator14/8  "V_BIAS"
  Demux11/6 -> Bus Creator14/6  "PSI_BIAS"
  Demux11/2 -> Bus Creator14/2  "Y_BIAS"
  Demux11/17 -> Bus Creator14/17  "WYD_BIAS"
  Demux11/14 -> Bus Creator14/14  "AY_BIAS"
  Demux11/10 -> Bus Creator14/10  "WX_BIAS"
  Demux11/16 -> Bus Creator14/16  "WXD_BIAS"

== system PX4_Run_Mode_R2017b/SENSOR_FILTER/Fixed Bias removal and scaling/Parameter Bus Creation/Kalman Filter ==
  A matrix : Subsystem
  B matrix : Subsystem
  Bus Creator1 : BusCreator  Inputs=4
  Bus Creator6 : BusCreator  Inputs=3
  Bus Creator9 : BusCreator  Inputs=8
  C matrix : Subsystem
  D matrix : Subsystem
  Data Type Conversion : DataTypeConversion  OutDataTypeStr=single
  Data Type Conversion1 : DataTypeConversion  OutDataTypeStr=single
  Demux1 : Demux
  Demux6 : Demux  Outputs=3
  Initialize Kalman Filter : MATLAB Function  TreatAsAtomicUnit=on
  Q matrix : Subsystem
  R matrix : Subsystem
  Kalman Filter Parameters Out : Outport
  wires:
  Bus Creator9/1 -> Kalman Filter Parameters Out/1  "Kalman Filter Parameters"
  Initialize Kalman Filter/7(pnvec) -> Data Type Conversion/1
  Demux6/1 -> Bus Creator6/1  "pn_x"
  Demux6/2 -> Bus Creator6/2  "pn_y"
  Bus Creator6/1 -> Bus Creator9/7  "pn vector"
  Initialize Kalman Filter/1(Amat) -> A matrix/1(A matrix In)
  A matrix/1(A matrix Out) -> Bus Creator9/1  "A matrix"
  Initialize Kalman Filter/2(Bmat) -> B matrix/1(B matrix In)
  B matrix/1(B matrix Out) -> Bus Creator9/2  "B matrix"
  C matrix/1(C matrix Out) -> Bus Creator9/3  "C matrix"
  Initialize Kalman Filter/3(Cmat) -> C matrix/1(C matrix In)
  Initialize Kalman Filter/4(Dmat) -> D matrix/1(D matrix In)
  D matrix/1(D matrix Out) -> Bus Creator9/4  "D matrix"
  Initialize Kalman Filter/5(Qmat) -> Q matrix/1(Q matrix In)
  Q matrix/1(Q matrix Out) -> Bus Creator9/5  "Q matrix"
  Initialize Kalman Filter/6(Rmat) -> R matrix/1(R matrix In)
  R matrix/1(R matrix Out) -> Bus Creator9/6  "R matrix"
  Demux6/3 -> Bus Creator6/3  "pn_z"
  Data Type Conversion/1 -> Demux6/1
  Demux1/1 -> Bus Creator1/1  "mn_x"
  Demux1/2 -> Bus Creator1/2  "mn_y"
  Bus Creator1/1 -> Bus Creator9/8  "mn vector"
  Demux1/3 -> Bus Creator1/3  "mn_z"
  Data Type Conversion1/1 -> Demux1/1
  Initialize Kalman Filter/8(mnvec) -> Data Type Conversion1/1
  Demux1/4 -> Bus Creator1/4  "m_son"

== system PX4_Run_Mode_R2017b/SENSOR_FILTER/Fixed Bias removal and scaling/Parameter Bus Creation/Madgewick Filter ==
  Bus Creator9 : BusCreator  Inputs=11
  Data Type Conversion : DataTypeConversion  OutDataTypeStr=single
  Demux : Demux  Outputs=11
  Initial Madgewick : MATLAB Function  TreatAsAtomicUnit=on
  Madgewick Filter Parameters Out : Outport
  wires:
  Bus Creator9/1 -> Madgewick Filter Parameters Out/1  "Madgewick Filter Parameters"
  Initial Madgewick/1(y) -> Data Type Conversion/1
  Demux/6 -> Bus Creator9/6  "thg_y"
  Demux/7 -> Bus Creator9/7  "thg_z"
  Demux/5 -> Bus Creator9/5  "thg_x"
  Demux/8 -> Bus Creator9/8  "m0"
  Demux/4 -> Bus Creator9/4  "Kapp"
  Demux/9 -> Bus Creator9/9  "Dip0"
  Demux/3 -> Bus Creator9/3  "app_z"
  Demux/10 -> Bus Creator9/10  "thdip"
  Demux/2 -> Bus Creator9/2  "app_y"
  Demux/11 -> Bus Creator9/11  "Beta"
  Demux/1 -> Bus Creator9/1  "app_x"
  Data Type Conversion/1 -> Demux/1

== system PX4_Run_Mode_R2017b/SENSOR_FILTER/Fixed Bias removal and scaling/Parameter Bus Creation/Magnetometer ==
  Parameters Magnetometer : Inport
  Bus Creator2 : BusCreator  Inputs=15
  Demux : Demux  Outputs=15
  Magnetometer Parameters Out : Outport
  wires:
  Parameters Magnetometer/1 -> Demux/1
  Demux/3 -> Bus Creator2/3  "CAL_MAG0_XZSCALE"
  Demux/5 -> Bus Creator2/5  "CAL_MAG0_YYSCALE"
  Demux/14 -> Bus Creator2/14  "CAL_MAG0_YCURCOR"
  Demux/8 -> Bus Creator2/8  "CAL_MAG0_ZYSCALE"
  Demux/10 -> Bus Creator2/10  "CAL_MAG0_XOFFSET"
  Demux/12 -> Bus Creator2/12  "CAL_MAG0_ZOFFSET"
  Demux/7 -> Bus Creator2/7  "CAL_MAG0_ZXSCALE"
  Demux/9 -> Bus Creator2/9  "CAL_MAG0_ZZSCALE"
  Demux/2 -> Bus Creator2/2  "CAL_MAG0_XYSCALE"
  Demux/15 -> Bus Creator2/15  "CAL_MAG0_ZCURCOR"
  Demux/6 -> Bus Creator2/6  "CAL_MAG0_YZSCALE"
  Demux/11 -> Bus Creator2/11  "CAL_MAG0_YOFFSET"
  Demux/13 -> Bus Creator2/13  "CAL_MAG0_XCURCOR"
  Demux/4 -> Bus Creator2/4  "CAL_MAG0_YXSCALE"
  Demux/1 -> Bus Creator2/1  "CAL_MAG0_XXSCALE"
  Bus Creator2/1 -> Magnetometer Parameters Out/1  "Magnetometer Parameters"

== system PX4_Run_Mode_R2017b/SENSOR_FILTER/Fixed Bias removal and scaling/Parameter Bus Creation/Motor Mixing ==
  Bus Creator13 : BusCreator  Inputs=16
  Constant45 : Constant  Value=T1  SampleTime=Ts
  Constant46 : Constant  Value=T2  SampleTime=Ts
  Constant47 : Constant  Value=T3  SampleTime=Ts
  Constant48 : Constant  Value=T4  SampleTime=Ts
  Constant49 : Constant  Value=R1  SampleTime=Ts
  Constant50 : Constant  Value=R2  SampleTime=Ts
  Constant51 : Constant  Value=R3  SampleTime=Ts
  Constant52 : Constant  Value=R4  SampleTime=Ts
  Constant53 : Constant  Value=P1  SampleTime=Ts
  Constant54 : Constant  Value=P2  SampleTime=Ts
  Constant55 : Constant  Value=P3  SampleTime=Ts
  Constant56 : Constant  Value=P4  SampleTime=Ts
  Constant57 : Constant  Value=Y1  SampleTime=Ts
  Constant58 : Constant  Value=Y2  SampleTime=Ts
  Constant59 : Constant  Value=Y3  SampleTime=Ts
  Constant60 : Constant  Value=Y4  SampleTime=Ts
  Motor Mixing Parameters Out : Outport
  wires:
  Constant45/1 -> Bus Creator13/1  "T1"
  Constant56/1 -> Bus Creator13/12  "P4"
  Constant54/1 -> Bus Creator13/10  "P2"
  Constant60/1 -> Bus Creator13/16  "Y4"
  Constant50/1 -> Bus Creator13/6  "R2"
  Constant51/1 -> Bus Creator13/7  "R3"
  Constant53/1 -> Bus Creator13/9  "P1"
  Constant52/1 -> Bus Creator13/8  "R4"
  Constant57/1 -> Bus Creator13/13  "Y1"
  Constant55/1 -> Bus Creator13/11  "P3"
  Constant46/1 -> Bus Creator13/2  "T2"
  Bus Creator13/1 -> Motor Mixing Parameters Out/1  "Motor Mixing Parameters"
  Constant48/1 -> Bus Creator13/4  "T4"
  Constant59/1 -> Bus Creator13/15  "Y3"
  Constant47/1 -> Bus Creator13/3  "T3"
  Constant58/1 -> Bus Creator13/14  "Y2"
  Constant49/1 -> Bus Creator13/5  "R1"

== system PX4_Run_Mode_R2017b/SENSOR_FILTER/Fixed Bias removal and scaling/Parameter Bus Creation/PWM ==
  Bus Creator12 : BusCreator  Inputs=4
  Constant41 : Constant  Value=PWM_a  SampleTime=Ts
  Constant42 : Constant  Value=PWM_b  SampleTime=Ts
  Constant43 : Constant  Value=PWM_c  SampleTime=Ts
  Constant44 : Constant  Value=PWM_d  SampleTime=Ts
  PWM Parameters Out : Outport
  wires:
  Constant41/1 -> Bus Creator12/1  "PWM_a"
  Constant44/1 -> Bus Creator12/4  "PWM_d"
  Constant42/1 -> Bus Creator12/2  "PWM_b"
  Bus Creator12/1 -> PWM Parameters Out/1  "PWM Parameters"
  Constant43/1 -> Bus Creator12/3  "PWM_c"

== system PX4_Run_Mode_R2017b/SENSOR_FILTER/Fixed Bias removal and scaling/Parameter Bus Creation/RC Parameters ==
  Bus Creator10 : BusCreator  Inputs=16
  Constant24 : Constant  Value=RC1_MIN  SampleTime=Ts
  Constant25 : Constant  Value=RC1_MAX  SampleTime=Ts
  Constant26 : Constant  Value=RC1_TRIM  SampleTime=Ts
  Constant27 : Constant  Value=RC1_DB  SampleTime=Ts
  Constant28 : Constant  Value=RC2_MIN  SampleTime=Ts
  Constant29 : Constant  Value=RC2_MAX  SampleTime=Ts
  Constant30 : Constant  Value=RC2_TRIM  SampleTime=Ts
  Constant31 : Constant  Value=RC2_DB  SampleTime=Ts
  Constant32 : Constant  Value=RC3_MIN  SampleTime=Ts
  Constant33 : Constant  Value=RC3_MAX  SampleTime=Ts
  Constant34 : Constant  Value=RC3_TRIM  SampleTime=Ts
  Constant35 : Constant  Value=RC3_DB  SampleTime=Ts
  Constant36 : Constant  Value=RC4_MIN  SampleTime=Ts
  Constant37 : Constant  Value=RC4_MAX  SampleTime=Ts
  Constant66 : Constant  Value=RC4_TRIM  SampleTime=Ts
  Constant67 : Constant  Value=RC4_DB  SampleTime=Ts
  RC Parameters Out : Outport
  wires:
  Constant27/1 -> Bus Creator10/4  "RC1_DB"
  Constant37/1 -> Bus Creator10/14  "RC4_MAX"
  Constant36/1 -> Bus Creator10/13  "RC4_MIN"
  Constant26/1 -> Bus Creator10/3  "RC1_TRIM"
  Constant33/1 -> Bus Creator10/10  "RC3_MAX"
  Constant66/1 -> Bus Creator10/15  "RC4_TRIM"
  Constant67/1 -> Bus Creator10/16  "RC4_DB"
  Constant34/1 -> Bus Creator10/11  "RC3_TRIM"
  Constant25/1 -> Bus Creator10/2  "RC1_MAX"
  Constant24/1 -> Bus Creator10/1  "RC1_MIN"
  Constant30/1 -> Bus Creator10/7  "RC2_TRIM"
  Constant31/1 -> Bus Creator10/8  "RC2_DB"
  Constant28/1 -> Bus Creator10/5  "RC2_MIN"
  Constant35/1 -> Bus Creator10/12  "RC3_DB"
  Bus Creator10/1 -> RC Parameters Out/1  "RC Parameters"
  Constant29/1 -> Bus Creator10/6  "RC2_MAX"
  Constant32/1 -> Bus Creator10/9  "RC3_MIN"

== system PX4_Run_Mode_R2017b/SENSOR_FILTER/Fixed Bias removal and scaling/Parameter Bus Creation/Sonar ==
  Parameters Sonar : Inport
  Bus Creator7 : BusCreator  Inputs=2
  Demux16 : Demux  Outputs=2
  Sonar Parameters Out : Outport
  wires:
  Demux16/2 -> Bus Creator7/2  "CAL_SONAR_OFFSET"
  Demux16/1 -> Bus Creator7/1  "CAL_SONAR_SCALE"
  Parameters Sonar/1 -> Demux16/1
  Bus Creator7/1 -> Sonar Parameters Out/1  "Sonar Parameters"

== system PX4_Run_Mode_R2017b/SENSOR_FILTER/Fixed Bias removal and scaling/Parameter Bus Creation/State Limit ==
  Bus Creator11 : BusCreator  Inputs=6
  Constant38 : Constant  Value=PITCH_MAX  SampleTime=Ts
  Constant39 : Constant  Value=ROLL_MAX  SampleTime=Ts
  Constant40 : Constant  Value=YAW_MAX  SampleTime=Ts
  Constant68 : Constant  Value=X_MAX  SampleTime=Ts
  Constant69 : Constant  Value=Y_MAX  SampleTime=Ts
  Constant70 : Constant  Value=Z_MAX  SampleTime=Ts
  State Limit Parameters Out : Outport
  wires:
  Constant69/1 -> Bus Creator11/5  "Y_MAX"
  Constant68/1 -> Bus Creator11/4  "X_MAX"
  Constant38/1 -> Bus Creator11/1  "PITCH_MAX"
  Bus Creator11/1 -> State Limit Parameters Out/1  "State Limit Parameters"
  Constant70/1 -> Bus Creator11/6  "Z_MAX"
  Constant39/1 -> Bus Creator11/2  "ROLL_MAX"
  Constant40/1 -> Bus Creator11/3  "YAW_MAX"

== system PX4_Run_Mode_R2017b/SENSOR_FILTER/Fixed Bias removal and scaling/Parameter Bus Creation/Kalman Filter/A matrix ==
  A matrix In : Inport
  Bus Creator : BusCreator  Inputs=36
  Data Type Conversion : DataTypeConversion  OutDataTypeStr=single
  Demux : Demux  Outputs=36
  A matrix Out : Outport
  wires:
  A matrix In/1 -> Data Type Conversion/1
  Bus Creator/1 -> A matrix Out/1  "A matrix"
  Demux/8 -> Bus Creator/8  "A22"
  Demux/10 -> Bus Creator/10  "A42"
  Demux/19 -> Bus Creator/19  "A14"
  Demux/5 -> Bus Creator/5  "A51"
  Demux/13 -> Bus Creator/13  "A13"
  Demux/20 -> Bus Creator/20  "A24"
  Demux/9 -> Bus Creator/9  "A32"
  Demux/18 -> Bus Creator/18  "A63"
  Demux/6 -> Bus Creator/6  "A61"
  Demux/12 -> Bus Creator/12  "A62"
  Demux/4 -> Bus Creator/4  "A41"
  Demux/7 -> Bus Creator/7  "A12"
  Demux/17 -> Bus Creator/17  "A53"
  Demux/11 -> Bus Creator/11  "A52"
  Demux/15 -> Bus Creator/15  "A33"
  Demux/3 -> Bus Creator/3  "A31"
  Demux/21 -> Bus Creator/21  "A34"
  Demux/14 -> Bus Creator/14  "A23"
  Demux/16 -> Bus Creator/16  "A43"
  Demux/34 -> Bus Creator/34  "A46"
  Demux/28 -> Bus Creator/28  "A45"
  Demux/30 -> Bus Creator/30  "A65"
  Demux/27 -> Bus Creator/27  "A35"
  Demux/29 -> Bus Creator/29  "A55"
  Demux/31 -> Bus Creator/31  "A16"
  Demux/32 -> Bus Creator/32  "A26"
  Demux/22 -> Bus Creator/22  "A44"
  Demux/24 -> Bus Creator/24  "A64"
  Demux/33 -> Bus Creator/33  "A36"
  Demux/23 -> Bus Creator/23  "A54"
  Demux/36 -> Bus Creator/36  "A66"
  Demux/25 -> Bus Creator/25  "A15"
  Demux/26 -> Bus Creator/26  "A25"
  Demux/35 -> Bus Creator/35  "A56"
  Demux/2 -> Bus Creator/2  "A21"
  Demux/1 -> Bus Creator/1  "A11"
  Data Type Conversion/1 -> Demux/1

== system PX4_Run_Mode_R2017b/SENSOR_FILTER/Fixed Bias removal and scaling/Parameter Bus Creation/Kalman Filter/B matrix ==
  B matrix In : Inport
  Bus Creator : BusCreator  Inputs=18
  Data Type Conversion : DataTypeConversion  OutDataTypeStr=single
  Demux : Demux  Outputs=18
  B matrix Out : Outport
  wires:
  B matrix In/1 -> Data Type Conversion/1
  Bus Creator/1 -> B matrix Out/1  "B matrix"
  Demux/8 -> Bus Creator/8  "B22"
  Demux/10 -> Bus Creator/10  "B42"
  Demux/5 -> Bus Creator/5  "B51"
  Demux/13 -> Bus Creator/13  "B13"
  Demux/9 -> Bus Creator/9  "B32"
  Demux/18 -> Bus Creator/18  "B63"
  Demux/6 -> Bus Creator/6  "B61"
  Demux/12 -> Bus Creator/12  "B62"
  Demux/4 -> Bus Creator/4  "B41"
  Demux/7 -> Bus Creator/7  "B12"
  Demux/17 -> Bus Creator/17  "B53"
  Demux/11 -> Bus Creator/11  "B52"
  Demux/15 -> Bus Creator/15  "B33"
  Demux/3 -> Bus Creator/3  "B31"
  Demux/14 -> Bus Creator/14  "B23"
  Demux/16 -> Bus Creator/16  "B43"
  Demux/2 -> Bus Creator/2  "B21"
  Demux/1 -> Bus Creator/1  "B11"
  Data Type Conversion/1 -> Demux/1
